simulink model "simple_walk_3d_with_feet"  (R2015a)
settings: Solver=ode23t  StartTime=0.0  StopTime=t_end  FixedStep=0.001
InitFcn:
  | colors
  | simulation_params
  | mechanical_params
StartFcn:
  | tic
StopFcn:
  | stopscript
values from neighbouring files (symbols this model uses):
  A_lpf_velocity = 1 + B1_lpf_velocity + B2_lpf_velocity    [simulation_params.m]
  ankle_stiffness = 1/2*pi    (= 1.57079632679)    [mechanical_params.m]
  B1_lpf_velocity = -2*exp(-lpf_damping*fcut_velocity*sample_time)*cos(fcut_velocity*sample_time*sqrt(1-lpf_damping^2))    [simulation_params.m]
  B2_lpf_velocity = exp(-2*lpf_damping*fcut_velocity*sample_time)    [simulation_params.m]
  b_hmotor = 0    [mechanical_params.m]
  b_leg_spring = 0.075*sqrt(k_leg_spring*0.5*.25^2)    [mechanical_params.m]
  b_rotor = 0*60/(2*pi)*9.725e-5    (= 0)    [mechanical_params.m]
  breakaway_friction = [25 25 25 25]    [mechanical_params.m]
  coulomb_friction = [20 20 20 20]    [mechanical_params.m]
  d_com = (d_hip_com_to_torso_com*m_torso)/(m_torso + num_legs*m_hshaft)    [mechanical_params.m]
  delta_phi_max = 160*pi/180    (= 2.79252680319)    [mechanical_params.m]
  delta_phi_min = 25.5*pi/180    (= 0.445058959259)    [mechanical_params.m]
  friction_linear_zone = [0.5 0.5 0.5 0.5].*pi/180    [mechanical_params.m]
  g = 9.81    [mechanical_params.m]
  HIP_MTR_MAX_TORQUE = max_current_hip*Kt_hip*N_h    (= 629.28)    [mechanical_params.m]
  initial_dx = 0    [mechanical_params.m]
  initial_hip_roll = -0.15    [mechanical_params.m]
  initial_pitch_joint_height = initial_com_height + boom_mount_to_com    [mechanical_params.m]
  initial_torso_pitch = 0*pi/180    (= 0)    [mechanical_params.m]
  initial_torso_roll = 0*pi/180    (= 0)    [mechanical_params.m]
  initial_torso_yaw = 0*pi/180    (= 0)    [mechanical_params.m]
  k_gx = m_total*g/0.005    (= 114164.30664)    [mechanical_params.m]
  k_gy = m_total*g/0.005    (= 114164.30664)    [mechanical_params.m]
  k_leg_spring = 2950    [mechanical_params.m]
  k_phi = 5000    [mechanical_params.m]
  Kb_leg = 0.121    [mechanical_params.m]
  Kt_leg = 0.121    [mechanical_params.m]
  L_leg = 0.102e-3    (= 0.000102)    [mechanical_params.m]
  l_lowerleg = 0.49    [mechanical_params.m]
  l_seg = 0.5    [mechanical_params.m]
  LEG_MTR_MAX_TORQUE = max_current_leg * Kt_leg * N    (= 1210)    [mechanical_params.m]
  lowerleg_12 = 0.40    (= 0.4)    [mechanical_params.m]
  m_fblink = 0.46    [mechanical_params.m]
  m_foot = 0.0857    [mechanical_params.m]
  m_hshaft = 18    [mechanical_params.m]
  m_lowerleg = 0.4438    [mechanical_params.m]
  m_output_gear = 1e-5    (= 1e-05)    [mechanical_params.m]
  m_rotor = 1e-5    (= 1e-05)    [mechanical_params.m]
  m_shin = 0.75    [mechanical_params.m]
  m_thigh = 0.69    [mechanical_params.m]
  m_torso = 17.5    [mechanical_params.m]
  m_total = num_legs*(m_hshaft + m_thigh + m_lowerleg + m_shin + m_fblink + 2*m_gearing) + m_torso    (= 58.18772)    [mechanical_params.m]
  m_virtual_gear = 1e-5    (= 1e-05)    [mechanical_params.m]
  max_current_leg = 200    [mechanical_params.m]
  max_voltage_leg = 50    [mechanical_params.m]
  mu_hmotor = 0.90    (= 0.9)    [mechanical_params.m]
  mu_motor = 0.85    [mechanical_params.m]
  mu_slide = 0.8    [mechanical_params.m]
  mu_stick = 0.9    [mechanical_params.m]
  N = 50    [mechanical_params.m]
  N_h = r_hip_shaft / r_hip_gearhead    (= 57)    [mechanical_params.m]
  output_sample_time = 1/30    (= 0.0333333333333)    [simulation_params.m]
  phi_max_collision = -5*pi/180    (= -0.0872664625997)    [mechanical_params.m]
  phi_roll_max = pi + 16*pi/180    (= 3.42084533391)    [mechanical_params.m]
  phi_roll_min = pi - 9*pi/180    (= 2.98451302091)    [mechanical_params.m]
  phi_shin_max = 3*pi/2 + 17.5*pi/180    (= 5.01782159948)    [mechanical_params.m]
  phi_shin_min = pi - 45*pi/180    (= 2.35619449019)    [mechanical_params.m]
  phi_thigh_max = pi + 45*pi/180    (= 3.92699081699)    [mechanical_params.m]
  phi_thigh_min = pi/2 - 17.5*pi/180    (= 1.2653637077)    [mechanical_params.m]
  r_hip_gearhead = 0.009525    [mechanical_params.m]
  r_hip_shaft = 0.542925    [mechanical_params.m]
  R_leg = 0.052    [mechanical_params.m]
  r_rotor = 0.001    [mechanical_params.m]
  r_virtual_gear = N*r_rotor    (= 0.05)    [mechanical_params.m]
  s = (clamp(f, tl, tu) - tl)/(tu - tl)    [controller.m]
  sample_time = 1/sample_freq    (= 0.001)    [simulation_params.m]
  shin_12 = 0.40    (= 0.4)    [mechanical_params.m]
  shin_initial_l = initial_l_leg_angle + acos(initial_l_leg_length)    [mechanical_params.m]
  shin_initial_r = initial_r_leg_angle + acos(initial_r_leg_length)    [mechanical_params.m]
  thigh_initial_l = initial_l_leg_angle - acos(initial_l_leg_length)    [mechanical_params.m]
  thigh_initial_r = initial_r_leg_angle - acos(initial_r_leg_length)    [mechanical_params.m]
  v_gx_max = 0.03    [mechanical_params.m]
  v_gy_max = 0.03    [mechanical_params.m]
  v_phi_max = 1/60    (= 0.0166666666667)    [mechanical_params.m]
  viscous_friction = [0.001 0.001 0.001 0.001]    [mechanical_params.m]
  vLimit = 0.01    [mechanical_params.m]
undefined symbols (not defined in the file or in its folder): fblink_color_d, floor_color_d, foot_color_d, hshaft_color_d, lowerleg_color_d, rad, sgn, shin_color_d, t_friction, thigh_color_d, torso_color_d, X, Y, Z
libraries: sm_lib x177, nesl_utility x130, simulink x57, fl_lib x16, simulink_extras x4, mblibv1 x2, commnoisgen2 x1, vrlib x1
(part 4 of 8)

== system simple_walk_3d_with_feet/Mechanical Simulation Layer/L Back Ground Contact/Ground Friction Model ==
  note: Normal Ground Stiction Model
  note: Transverse Ground Friction Model
  delta normal [m] : Inport
  vnormal [m/s] : Inport  Port=2
  x [m] : Inport  Port=3
  vx [m/s] : Inport  Port=4
  y [m] : Inport  Port=5
  vy [m/s] : Inport  Port=6
  Contact! : EnablePort  StatesWhenEnabling=reset
  Data Type Conversion : DataTypeConversion  OutDataTypeStr=double
  Friction Switch : Subsystem
  Gain3 : Gain  Gain=k_gy
  Gain4 : Gain  Gain=1/v_gy_max
  Logical Operator : Logic  Operator=NOT  AllPortsSameDT=off  OutDataTypeStr=boolean
  Mux1 : Mux  Inputs=2
  Sum1 : Sum
  Sum2 : Sum
  normal-Axis Ground Force : Fcn  Expr="- u(1)  *  (1-u(2)) * (u(2)<1)"
  t-Axis Kinetic Friction Model : Subsystem
  t-Axis Static Friction Model : Subsystem
  FxFriction [N] : Outport  OutputWhenDisabled=reset  InitialOutput=0
      settings: AttributesFormatString=initial = '%<InitialOutput>'\nwhen\ndisabled\n'%<OutputWhenDisabled>'
  FyFriction [N] : Outport  Port=2  OutputWhenDisabled=reset  InitialOutput=0
      settings: AttributesFormatString=initial = '%<InitialOutput>'\nwhen\ndisabled\n'%<OutputWhenDisabled>'
  Fn_Ground[N] : Outport  Port=3  OutputWhenDisabled=reset  InitialOutput=0
      settings: AttributesFormatString=initial = '%<InitialOutput>'\nwhen disabled = '%<OutputWhenDisabled>'
  Stiction! : Outport  Port=4  OutputWhenDisabled=reset  InitialOutput=0
      settings: AttributesFormatString=initial = '%<InitialOutput>'\nwhen\ndisabled\n'%<OutputWhenDisabled>'
  wires:
  Data Type Conversion/1 -> Stiction!/1
  vy [m/s]/1 -> t-Axis Static Friction Model/5(vel_y [m/s]), t-Axis Kinetic Friction Model/4(vel_y [m/s])
  y [m]/1 -> t-Axis Kinetic Friction Model/3(pos_y [m]), t-Axis Static Friction Model/4(pos_y [m])
  t-Axis Kinetic Friction Model/2(posFP_y [m]) -> t-Axis Static Friction Model/7(posFP_y [m])
  Sum2/1 -> FyFriction [N]/1
  t-Axis Kinetic Friction Model/5(Fy_Slide [N]) -> Sum2/2
  t-Axis Static Friction Model/1(Fy_Stick [N]) -> Sum2/1
  Gain4/1 -> Mux1/2
  Gain3/1 -> Mux1/1
  Mux1/1 -> normal-Axis Ground Force/1
  Logical Operator/1 -> t-Axis Kinetic Friction Model/Enable
  t-Axis Kinetic Friction Model/3(Stiction!) -> Friction Switch/2(Stick!)
  t-Axis Static Friction Model/3(Sliding!) -> Friction Switch/1(Slide!)
  Friction Switch/1(Stiction) -> t-Axis Static Friction Model/Enable, Logical Operator/1, Data Type Conversion/1
  Sum1/1 -> FxFriction [N]/1
  t-Axis Static Friction Model/2(Fx_Stick [N]) -> Sum1/1
  t-Axis Kinetic Friction Model/4(Fx_Slide [N]) -> Sum1/2
  t-Axis Kinetic Friction Model/1(posFP_x [m]) -> t-Axis Static Friction Model/6(posFP_x [m])
  vx [m/s]/1 -> t-Axis Static Friction Model/3(vel_x [m/s]), t-Axis Kinetic Friction Model/2(vel_x [m/s])
  x [m]/1 -> t-Axis Static Friction Model/2(pos_x [m]), t-Axis Kinetic Friction Model/1(pos_x [m])
  vnormal [m/s]/1 -> Gain4/1
  delta normal [m]/1 -> Gain3/1
  normal-Axis Ground Force/1 -> Fn_Ground[N]/1, t-Axis Kinetic Friction Model/5(F_Normal [N]), t-Axis Static Friction Model/1(F_Normal [N])

== system simple_walk_3d_with_feet/Mechanical Simulation Layer/L Front Ground Contact/Ground Friction Model ==
  note: Transverse Ground Friction Model
  note: Normal Ground Stiction Model
  delta normal [m] : Inport
  vnormal [m/s] : Inport  Port=2
  x [m] : Inport  Port=3
  vx [m/s] : Inport  Port=4
  y [m] : Inport  Port=5
  vy [m/s] : Inport  Port=6
  Contact! : EnablePort  StatesWhenEnabling=reset
  Data Type Conversion : DataTypeConversion  OutDataTypeStr=double
  Friction Switch : Subsystem
  Gain3 : Gain  Gain=k_gy
  Gain4 : Gain  Gain=1/v_gy_max
  Logical Operator : Logic  Operator=NOT  AllPortsSameDT=off  OutDataTypeStr=boolean
  Mux1 : Mux  Inputs=2
  Sum1 : Sum
  Sum2 : Sum
  normal-Axis Ground Force : Fcn  Expr="- u(1)  *  (1-u(2)) * (u(2)<1)"
  t-Axis Kinetic Friction Model : Subsystem
  t-Axis Static Friction Model : Subsystem
  FxFriction [N] : Outport  OutputWhenDisabled=reset  InitialOutput=0
      settings: AttributesFormatString=initial = '%<InitialOutput>'\nwhen\ndisabled\n'%<OutputWhenDisabled>'
  FyFriction [N] : Outport  Port=2  OutputWhenDisabled=reset  InitialOutput=0
      settings: AttributesFormatString=initial = '%<InitialOutput>'\nwhen\ndisabled\n'%<OutputWhenDisabled>'
  Fn_Ground[N] : Outport  Port=3  OutputWhenDisabled=reset  InitialOutput=0
      settings: AttributesFormatString=initial = '%<InitialOutput>'\nwhen disabled = '%<OutputWhenDisabled>'
  Stiction! : Outport  Port=4  OutputWhenDisabled=reset  InitialOutput=0
      settings: AttributesFormatString=initial = '%<InitialOutput>'\nwhen\ndisabled\n'%<OutputWhenDisabled>'
  wires:
  normal-Axis Ground Force/1 -> t-Axis Static Friction Model/1(F_Normal [N]), t-Axis Kinetic Friction Model/5(F_Normal [N]), Fn_Ground[N]/1
  delta normal [m]/1 -> Gain3/1
  vnormal [m/s]/1 -> Gain4/1
  x [m]/1 -> t-Axis Kinetic Friction Model/1(pos_x [m]), t-Axis Static Friction Model/2(pos_x [m])
  vx [m/s]/1 -> t-Axis Kinetic Friction Model/2(vel_x [m/s]), t-Axis Static Friction Model/3(vel_x [m/s])
  t-Axis Kinetic Friction Model/1(posFP_x [m]) -> t-Axis Static Friction Model/6(posFP_x [m])
  t-Axis Kinetic Friction Model/4(Fx_Slide [N]) -> Sum1/2
  t-Axis Static Friction Model/2(Fx_Stick [N]) -> Sum1/1
  Sum1/1 -> FxFriction [N]/1
  Friction Switch/1(Stiction) -> Data Type Conversion/1, Logical Operator/1, t-Axis Static Friction Model/Enable
  t-Axis Static Friction Model/3(Sliding!) -> Friction Switch/1(Slide!)
  t-Axis Kinetic Friction Model/3(Stiction!) -> Friction Switch/2(Stick!)
  Logical Operator/1 -> t-Axis Kinetic Friction Model/Enable
  Mux1/1 -> normal-Axis Ground Force/1
  Gain3/1 -> Mux1/1
  Gain4/1 -> Mux1/2
  t-Axis Static Friction Model/1(Fy_Stick [N]) -> Sum2/1
  t-Axis Kinetic Friction Model/5(Fy_Slide [N]) -> Sum2/2
  Sum2/1 -> FyFriction [N]/1
  t-Axis Kinetic Friction Model/2(posFP_y [m]) -> t-Axis Static Friction Model/7(posFP_y [m])
  y [m]/1 -> t-Axis Static Friction Model/4(pos_y [m]), t-Axis Kinetic Friction Model/3(pos_y [m])
  vy [m/s]/1 -> t-Axis Kinetic Friction Model/4(vel_y [m/s]), t-Axis Static Friction Model/5(vel_y [m/s])
  Data Type Conversion/1 -> Stiction!/1

== system simple_walk_3d_with_feet/Mechanical Simulation Layer/L Hip Shaft/Frame Data ==
  Kinematic Data : ToWorkspace  VariableName=l_hip_out  SampleTime=output_sample_time
      settings: Save2DSignal=2-D array (concatenate along first dimension)
  Mux : Mux
  PS-Simulink Converter{,1..3} (4 alike) : nesl_utility/PS-Simulink Converter  PhysicalDomain=network_engine_domain  SubClassName=ps_output  LeftPortType=input  RightPortType=output  PseudoPeriodic=off  Frequencies=[]  Unit=1  AffineConversion=off
  Transform Sensor : sm_lib/Frames and Transforms/Transform Sensor  MeasurementFrame=World  SenseAngle=off  SenseAxis=off  SenseAngle1=off  SenseAngle2=off  SenseAngle3=off  SenseQ=on  SenseR=off  SenseOmegaX=off  SenseOmegaY=off  SenseOmegaZ=off  SenseOmega1=off  SenseOmega2=off  SenseOmega3=off  SenseQDot=off  SenseRDot=off  SenseAlphaX=off  SenseAlphaY=off  SenseAlphaZ=off  SenseAlpha1=off  SenseAlpha2=off  SenseAlpha3=off  SenseQDDot=off  SenseRDDot=off  SenseX=on  SenseY=on  SenseZ=on  SenseRad=off  SenseAzim=off  SenseDist=off  SenseInc=off  SenseXDot=off  SenseYDot=off  SenseZDot=off  SenseRadDot=off  SenseAzimDot=off  SenseDistDot=off  SenseIncDot=off  SenseXDDot=off  SenseYDDot=off  SenseZDDot=off  SenseRadDDot=off  SenseAzimDDot=off  SenseDistDDot=off  SenseIncDDot=off  BlockFunction=simmechanics.library.frames_transforms.transform_sensor
  World Frame : sm_lib/Frames and Transforms/World Frame  BlockFunction=simmechanics.library.frames_transforms.world_frame
  Frame : PMIOPort  Port=1  Side=Left
  wires:
  Mux/1 -> Kinematic Data/1
  PS-Simulink Converter/1 -> Mux/1
  PS-Simulink Converter1/1 -> Mux/2
  PS-Simulink Converter2/1 -> Mux/3
  PS-Simulink Converter3/1 -> Mux/4
  connections:
  PS-Simulink Converter3/LConn1 -- Transform Sensor/RConn5
  PS-Simulink Converter2/LConn1 -- Transform Sensor/RConn4
  PS-Simulink Converter1/LConn1 -- Transform Sensor/RConn3
  PS-Simulink Converter/LConn1 -- Transform Sensor/RConn2
  Transform Sensor/RConn1 -- Frame/RConn1
  Transform Sensor/LConn1 -- World Frame/RConn1

== system simple_walk_3d_with_feet/Mechanical Simulation Layer/L Leg/Angle Range Map ==
  "[-pi, pi]" : Inport
  Constant : Constant  Value=2*pi
  Sum3 : Sum  Inputs=|++
  Switch : Switch  ZeroCross=off
  "[0,2*pi]" : Outport
  wires:
  "[-pi, pi]"/1 -> Sum3/1, Switch/1, Switch/2
  Sum3/1 -> Switch/3
  Constant/1 -> Sum3/2
  Switch/1 -> "[0,2*pi]"/1

== system simple_walk_3d_with_feet/Mechanical Simulation Layer/L Leg/Angle Range Map1 ==
  "[-pi, pi]" : Inport
  Constant : Constant  Value=2*pi
  Sum3 : Sum  Inputs=|++
  Switch : Switch  ZeroCross=off
  "[0,2*pi]" : Outport
  wires:
  Switch/1 -> "[0,2*pi]"/1
  Constant/1 -> Sum3/2
  Sum3/1 -> Switch/3
  "[-pi, pi]"/1 -> Switch/2, Switch/1, Sum3/1

== system simple_walk_3d_with_feet/Mechanical Simulation Layer/L Leg/Four Bar Link ==
  CS1 to CS2 : sm_lib/Frames and Transforms/Rigid Transform  TranslationMethod=Cartesian  TranslationLengthUnit=m  TranslationStandardAxis=+Z  TranslationStandardOffset=0  TranslationCartesianOffset=[0 -l_seg 0]  TranslationROffset=0  TranslationROffsetUnits=m  TranslationZOffset=0  TranslationZOffsetUnits=m  TranslationThetaOffset=0  TranslationThetaOffsetUnits=deg  RotationMethod=None  RotationAngleUnits=deg  RotationStandardAxis=+Z  RotationAngle=0  RotationArbitraryAxis=[0 0 1]  FollAlignAxisA=+X  BaseAlignAxisA=+Y  FollAlignAxisB=+Y  BaseAlignAxisB=+Z  RotationMatrix=[1 0 0; 0 1 0; 0 0 1]  BlockFunction=simmechanics.library.frames_transforms.rigid_transform
  Frame Data : Subsystem
  Solid : sm_lib/Body Elements/Solid  InertiaType=Custom  Mass=m_fblink  MassUnits=kg  CenterOfMass=com_fblink  CenterOfMassUnits=m  MomentsOfInertia=i_fblink_moments  MomentsOfInertiaUnits=kg*m^2  ProductsOfInertia=i_fblink_products  ProductsOfInertiaUnits=kg*m^2  DensityBased=on  Density=1000  DensityUnits=kg/(m^3)  GraphicType=FromGeometry  MarkerShape=Sphere  MarkerSize=10  MarkerSizeUnits=m  GraphicVisPropType=AdvancedVisualProperties  GraphicDiffuseColor=fblink_color_d  GraphicSpecularColor=[1 1 1 1]  GraphicAmbientColor=[fblink_color_d/2 1]  GraphicEmissiveColor=[0 0 0 1]  GraphicShininess=128  GraphicOpacity=1.0  GeometryShape=FromFile  RectangleSize=[1 1]  RectangleSizeUnits=m  BrickDimensions=[0.1 l_seg 0.1]  BrickDimensionUnits=m  CylinderRadius=l_rad  CylinderRadiusUnits=m  CylinderLength=l_seg  CylinderLengthUnits=m  SphereRadius=1  SphereRadiusUnits=m  EllipsoidRadii=[1 1 1]  EllipsoidRadiiUnits=m  ExtrusionCrossSection=[1 1; -1 1; -1 -1; 1 -1]  ExtrusionCrossSectionUnits=m  ExtrusionLength=1  ExtrusionLengthUnits=m  PolygonNumSides=3  PolygonOuterRadius=1  PolygonOuterRadiusUnits=m  ExtGeomFileType=STL  ExtGeomFileName=four_bar_link.stl  ExtGeomFileUnits=m  RevolutionCrossSection=[1 1; 1 -1; 2 -1; 2 1]  RevolutionCrossSectionUnits=m  RevolutionExtent=Full  RevolutionAngle=180  RevolutionAngleUnits=deg  BlockFunction=simmechanics.library.body_elements.solid
  CS1 : PMIOPort  Port=1  Side=Left
  CS2 : PMIOPort  Port=2  Side=Right
  connections:
  CS2/RConn1 -- CS1 to CS2/RConn1
  Solid/RConn1 -- CS1/RConn1 -- Frame Data/LConn1 -- CS1 to CS2/LConn1

== system simple_walk_3d_with_feet/Mechanical Simulation Layer/L Leg/Lower Leg ==
  CS1 to CS2 : sm_lib/Frames and Transforms/Rigid Transform  TranslationMethod=Cartesian  TranslationLengthUnit=m  TranslationStandardAxis=+Z  TranslationStandardOffset=0  TranslationCartesianOffset=[0 -lowerleg_12 0]  TranslationROffset=0  TranslationROffsetUnits=m  TranslationZOffset=0  TranslationZOffsetUnits=m  TranslationThetaOffset=0  TranslationThetaOffsetUnits=deg  RotationMethod=None  RotationAngleUnits=deg  RotationStandardAxis=+Z  RotationAngle=45  RotationArbitraryAxis=[0 0 1]  FollAlignAxisA=+X  BaseAlignAxisA=+Y  FollAlignAxisB=+Y  BaseAlignAxisB=+Z  RotationMatrix=[1 0 0; 0 1 0; 0 0 1]  BlockFunction=simmechanics.library.frames_transforms.rigid_transform
  CS1 to CS3 : sm_lib/Frames and Transforms/Rigid Transform  TranslationMethod=Cartesian  TranslationLengthUnit=m  TranslationStandardAxis=+Z  TranslationStandardOffset=0  TranslationCartesianOffset=[0 -l_lowerleg 0]  TranslationROffset=0  TranslationROffsetUnits=m  TranslationZOffset=0  TranslationZOffsetUnits=m  TranslationThetaOffset=0  TranslationThetaOffsetUnits=deg  RotationMethod=None  RotationAngleUnits=deg  RotationStandardAxis=+Y  RotationAngle=-20  RotationArbitraryAxis=[0 0 1]  FollAlignAxisA=+X  BaseAlignAxisA=+Y  FollAlignAxisB=+Y  BaseAlignAxisB=+Z  RotationMatrix=[1 0 0; 0 1 0; 0 0 1]  BlockFunction=simmechanics.library.frames_transforms.rigid_transform
  Frame Data : Subsystem
  Solid : sm_lib/Body Elements/Solid  InertiaType=Custom  Mass=m_lowerleg  MassUnits=kg  CenterOfMass=com_lowerleg  CenterOfMassUnits=m  MomentsOfInertia=i_lowerleg_moments  MomentsOfInertiaUnits=kg*m^2  ProductsOfInertia=i_lowerleg_products  ProductsOfInertiaUnits=kg*m^2  DensityBased=on  Density=1000  DensityUnits=kg/(m^3)  GraphicType=FromGeometry  MarkerShape=Sphere  MarkerSize=10  MarkerSizeUnits=m  GraphicVisPropType=AdvancedVisualProperties  GraphicDiffuseColor=lowerleg_color_d  GraphicSpecularColor=[1 1 1 1]  GraphicAmbientColor=[lowerleg_color_d/2 1]  GraphicEmissiveColor=[0 0 0 1]  GraphicShininess=128  GraphicOpacity=1.0  GeometryShape=FromFile  RectangleSize=[1 1]  RectangleSizeUnits=m  BrickDimensions=[0.1 l_seg 0.1]  BrickDimensionUnits=m  CylinderRadius=l_rad  CylinderRadiusUnits=m  CylinderLength=l_seg  CylinderLengthUnits=m  SphereRadius=1  SphereRadiusUnits=m  EllipsoidRadii=[1 1 1]  EllipsoidRadiiUnits=m  ExtrusionCrossSection=[1 1; -1 1; -1 -1; 1 -1]  ExtrusionCrossSectionUnits=m  ExtrusionLength=1  ExtrusionLengthUnits=m  PolygonNumSides=3  PolygonOuterRadius=1  PolygonOuterRadiusUnits=m  ExtGeomFileType=STL  ExtGeomFileName=lower_leg_two_point.stl  ExtGeomFileUnits=m  RevolutionCrossSection=[1 1; 1 -1; 2 -1; 2 1]  RevolutionCrossSectionUnits=m  RevolutionExtent=Full  RevolutionAngle=180  RevolutionAngleUnits=deg  BlockFunction=simmechanics.library.body_elements.solid
  CS1 : PMIOPort  Port=1  Side=Left
  CS2 : PMIOPort  Port=2  Side=Right
  CS3 : PMIOPort  Port=3  Side=Right
  connections:
  CS3/RConn1 -- CS1 to CS3/RConn1
  Frame Data/LConn1 -- CS1 to CS3/LConn1 -- CS1 to CS2/LConn1 -- Solid/RConn1 -- CS1/RConn1
  CS2/RConn1 -- CS1 to CS2/RConn1

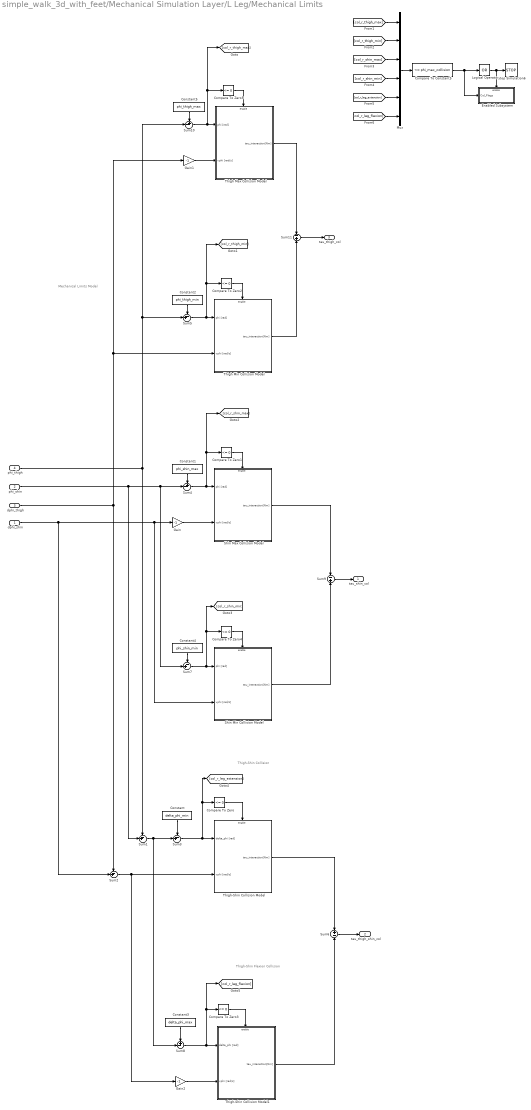
== system simple_walk_3d_with_feet/Mechanical Simulation Layer/L Leg/Mechanical Limits ==
  note: Thigh-Shin Flexion Collision
  note: Thigh-Shin Collision
  note: Mechanical Limits Model
  dphi_shin : Inport
  phi_shin : Inport  Port=2
  dphi_thigh : Inport  Port=3
  phi_thigh : Inport  Port=4
  Compare To Constant5 : simulink/Logic and Bit Operations/Compare To Constant  relop=<=  const=phi_max_collision  OutDataTypeStr=boolean  ZeroCross=off
  Compare To Zero{,1..5} (6 alike) : simulink/Logic and Bit Operations/Compare To Zero  relop=<=  OutDataTypeStr=boolean  ZeroCross=off
  Constant : Constant  Value=delta_phi_min
  Constant1 : Constant  Value=phi_shin_max
  Constant2 : Constant  Value=phi_thigh_min
  Constant3 : Constant  Value=delta_phi_max
  Constant4 : Constant  Value=phi_shin_min
  Constant5 : Constant  Value=phi_thigh_max
  Enabled Subsystem : Subsystem  TreatAsAtomicUnit=on
  Gain : Gain  Gain=-1
  Gain1 : Gain  Gain=-1
  Gain2 : Gain  Gain=-1
  Logical Operator : Logic  Operator=OR  Inputs=1  AllPortsSameDT=off  OutDataTypeStr=boolean
  Mux : Mux  Inputs=6
  Shin Max Collision Model : Subsystem
  Shin Min Collision Model : Subsystem
  Stop Simulation6 : Stop
  Sum{1..3,5,7} (5 alike) : Sum  Inputs=-+|
  Sum10 : Sum  Inputs=+-|
  Sum11 : Sum  Inputs=-|+
  Sum4 : Sum  Inputs=+-|
  Sum6 : Sum  Inputs=+|-
  Sum8 : Sum  Inputs=+-|
  Sum9 : Sum  Inputs=-|+
  Thigh Max Collision Model : Subsystem
  Thigh Min Collision Model : Subsystem
  Thigh-Shin Collision Model : Subsystem
  Thigh-Shin Collision Model1 : Subsystem
  tau_shin_col : Outport
  tau_thigh_shin_col : Outport  Port=2
  tau_thigh_col : Outport  Port=3
  wires:
  Compare To Constant5/1 -> Logical Operator/1, Enabled Subsystem/1(Col_Flags)
  Sum4/1 -> Shin Max Collision Model/1(phi [rad]), Compare To Zero1/1, [col_r_shin_max]
  Sum10/1 -> [col_r_thigh_max], Compare To Zero5/1, Thigh Max Collision Model/1(phi [rad])
  Logical Operator/1 -> Enabled Subsystem/Enable, Stop Simulation6/1
  Mux/1 -> Compare To Constant5/1
  [col_r_leg_flexion] -> Mux/6
  [col_r_leg_extension] -> Mux/5
  [col_r_shin_min] -> Mux/4
  [col_r_shin_max] -> Mux/3
  [col_r_thigh_min] -> Mux/2
  [col_r_thigh_max] -> Mux/1
  Thigh Max Collision Model/1(tau_interaction[Nm]) -> Sum11/1
  Gain1/1 -> Thigh Max Collision Model/2(vphi [rad/s])
  Thigh Min Collision Model/1(tau_interaction[Nm]) -> Sum11/2
  Sum11/1 -> tau_thigh_col/1
  Compare To Zero5/1 -> Thigh Max Collision Model/Enable
  Constant5/1 -> Sum10/1
  Sum6/1 -> tau_thigh_shin_col/1
  Shin Min Collision Model/1(tau_interaction[Nm]) -> Sum9/2
  Shin Max Collision Model/1(tau_interaction[Nm]) -> Sum9/1
  Sum9/1 -> tau_shin_col/1
  dphi_shin/1 -> Shin Min Collision Model/2(vphi [rad/s]), Gain/1, Sum2/2
  Sum7/1 -> Shin Min Collision Model/1(phi [rad]), Compare To Zero4/1, [col_r_shin_min]
  Constant4/1 -> Sum7/1
  Compare To Zero4/1 -> Shin Min Collision Model/Enable
  Gain2/1 -> Thigh-Shin Collision Model1/2(vphi [rad/s])
  Thigh-Shin Collision Model1/1(tau_interaction[Nm]) -> Sum6/2
  Thigh-Shin Collision Model/1(tau_interaction[Nm]) -> Sum6/1
  Sum8/1 -> Thigh-Shin Collision Model1/1(delta_phi [rad]), Compare To Zero3/1, [col_r_leg_flexion]
  Constant3/1 -> Sum8/1
  Compare To Zero3/1 -> Thigh-Shin Collision Model1/Enable
  Compare To Zero2/1 -> Thigh Min Collision Model/Enable
  Gain/1 -> Shin Max Collision Model/2(vphi [rad/s])
  Sum5/1 -> Thigh Min Collision Model/1(phi [rad]), Compare To Zero2/1, [col_r_thigh_min]
  Constant2/1 -> Sum5/1
  dphi_thigh/1 -> Sum2/1, Gain1/1, Thigh Min Collision Model/2(vphi [rad/s])
  phi_thigh/1 -> Sum1/1, Sum5/2, Sum10/2
  Constant1/1 -> Sum4/1
  Compare To Zero1/1 -> Shin Max Collision Model/Enable
  Sum3/1 -> Thigh-Shin Collision Model/1(delta_phi [rad]), Compare To Zero/1, [col_r_leg_extension]
  Constant/1 -> Sum3/1
  Sum2/1 -> Thigh-Shin Collision Model/2(vphi [rad/s]), Gain2/1
  phi_shin/1 -> Sum4/2, Sum7/2, Sum1/2
  Sum1/1 -> Sum3/2, Sum8/2
  Compare To Zero/1 -> Thigh-Shin Collision Model/Enable

== system simple_walk_3d_with_feet/Mechanical Simulation Layer/L Leg/Shin ==
  CS1 to CS2 : sm_lib/Frames and Transforms/Rigid Transform  TranslationMethod=Cartesian  TranslationLengthUnit=m  TranslationStandardAxis=+Z  TranslationStandardOffset=0  TranslationCartesianOffset=[0 -shin_12 0]  TranslationROffset=0  TranslationROffsetUnits=m  TranslationZOffset=0  TranslationZOffsetUnits=m  TranslationThetaOffset=0  TranslationThetaOffsetUnits=deg  RotationMethod=None  RotationAngleUnits=deg  RotationStandardAxis=+Z  RotationAngle=0  RotationArbitraryAxis=[0 0 1]  FollAlignAxisA=+X  BaseAlignAxisA=+Y  FollAlignAxisB=+Y  BaseAlignAxisB=+Z  RotationMatrix=[1 0 0; 0 1 0; 0 0 1]  BlockFunction=simmechanics.library.frames_transforms.rigid_transform
  Frame Data : Subsystem
  Solid : sm_lib/Body Elements/Solid  InertiaType=Custom  Mass=m_shin  MassUnits=kg  CenterOfMass=com_shin  CenterOfMassUnits=m  MomentsOfInertia=i_shin_moments  MomentsOfInertiaUnits=kg*m^2  ProductsOfInertia=i_shin_products  ProductsOfInertiaUnits=kg*m^2  DensityBased=on  Density=1000  DensityUnits=kg/(m^3)  GraphicType=FromGeometry  MarkerShape=Sphere  MarkerSize=10  MarkerSizeUnits=m  GraphicVisPropType=AdvancedVisualProperties  GraphicDiffuseColor=shin_color_d  GraphicSpecularColor=[1 1 1 1]  GraphicAmbientColor=[shin_color_d/2 1]  GraphicEmissiveColor=[0 0 0 1]  GraphicShininess=128  GraphicOpacity=1.0  GeometryShape=FromFile  RectangleSize=[1 1]  RectangleSizeUnits=m  BrickDimensions=[1 1 1]  BrickDimensionUnits=m  CylinderRadius=l_rad  CylinderRadiusUnits=m  CylinderLength=l_seg  CylinderLengthUnits=m  SphereRadius=1  SphereRadiusUnits=m  EllipsoidRadii=[1 1 1]  EllipsoidRadiiUnits=m  ExtrusionCrossSection=[1 1; -1 1; -1 -1; 1 -1]  ExtrusionCrossSectionUnits=m  ExtrusionLength=1  ExtrusionLengthUnits=m  PolygonNumSides=3  PolygonOuterRadius=1  PolygonOuterRadiusUnits=m  ExtGeomFileType=STL  ExtGeomFileName=shin.stl  ExtGeomFileUnits=m  RevolutionCrossSection=[1 1; 1 -1; 2 -1; 2 1]  RevolutionCrossSectionUnits=m  RevolutionExtent=Full  RevolutionAngle=180  RevolutionAngleUnits=deg  BlockFunction=simmechanics.library.body_elements.solid
  CS1 : PMIOPort  Port=1  Side=Left
  CS2 : PMIOPort  Port=2  Side=Right
  connections:
  CS1 to CS2/LConn1 -- CS1/RConn1 -- Frame Data/LConn1 -- Solid/RConn1
  CS2/RConn1 -- CS1 to CS2/RConn1

== system simple_walk_3d_with_feet/Mechanical Simulation Layer/L Leg/Shin SEA ==
  note: Shin SEA Mechanics
  Shin Gear Torque [Nm] : Inport
  Shin Joint [rad rad/s] : Inport  Port=2
  Demux : Demux  Outputs=2
  Gain : Gain  Gain=k_leg_spring
  Gain1 : Gain  Gain=b_leg_spring
  Initial Gear Angle : Constant  Value=shin_initial_l
  Inverse Gear Ratio2 : Gain  Gain=1/N
  Inverse Gear Ratio3 : Gain  Gain=Kt_leg
  Inverse Gear Ratio4 : Gain  Gain=1/Kt_leg
  Motor Efficiency : Gain  Gain=mu_motor
  Motor Controller : Subsystem  Commented=on
  Motor Electromagnetism : Subsystem  Commented=on
  Rotor Damping : Gain  Gain=b_rotor
  Rotor and Gearing : Subsystem
  Sum : Sum  Inputs=++|
  Sum2 : Sum  Inputs=+|-
  Sum3 : Sum  Inputs=|+-
  Sum4 : Sum  Inputs=+|-
  Sum5 : Sum  Inputs=|++
  Torque Limiter (outside) 2 : Saturate  UpperLimit=LEG_MTR_MAX_TORQUE  LowerLimit=-LEG_MTR_MAX_TORQUE  ZeroCross=off
      settings: AttributesFormatString=Hi: %<UpperLimit>\nLo: %<LowerLimit>
  Rotor Joint Conn : PMIOPort  Port=1  Side=Left
  Shin Joint Torque [Nm] : Outport
  Shin Gear [rad] : Outport  Port=2
  wires:
  Sum2/1 -> Gain/1
  Sum5/1 -> Rotor and Gearing/2(Spring Torque [Nm]), Shin Joint Torque [Nm]/1
  Sum3/1 -> Motor Efficiency/1
  Rotor Damping/1 -> Sum3/2
  Gain/1 -> Sum5/1  "tau_load"
  Gain1/1 -> Sum5/2
  Sum4/1 -> Gain1/1
  Shin Joint [rad rad/s]/1 -> Demux/1
  Demux/1 -> Sum2/2
  Demux/2 -> Sum4/2
  Inverse Gear Ratio3/1 -> Sum3/1
  Initial Gear Angle/1 -> Sum/1
  Sum/1 -> Shin Gear [rad]/1, Sum2/1
  Rotor and Gearing/1(Gearhead Position [rad]) -> Sum/2
  Rotor and Gearing/2(Gearhead Velocity [rad/s]) -> Sum4/1
  Motor Efficiency/1 -> Rotor and Gearing/1(Rotor Torque [Nm])
  Inverse Gear Ratio4/1 -> Inverse Gear Ratio3/1
  Motor Controller/1(Voltage [V]) -> Motor Electromagnetism/1(Voltage [V])
  Motor Electromagnetism/1(Current [A]) -> Motor Controller/2(Measured Current [A])
  Shin Gear Torque [Nm]/1 -> Torque Limiter (outside) 2/1
  Inverse Gear Ratio2/1 -> Inverse Gear Ratio4/1
  Rotor and Gearing/3(Rotor Velocity [rad/s]) -> Rotor Damping/1
  Torque Limiter (outside) 2/1 -> Inverse Gear Ratio2/1
  connections:
  Rotor and Gearing/LConn1 -- Rotor Joint Conn/RConn1

== system simple_walk_3d_with_feet/Mechanical Simulation Layer/L Leg/Thigh ==
  CS1 to CS2 : sm_lib/Frames and Transforms/Rigid Transform  TranslationMethod=Cartesian  TranslationLengthUnit=m  TranslationStandardAxis=+Z  TranslationStandardOffset=0  TranslationCartesianOffset=[0 -l_seg 0]  TranslationROffset=0  TranslationROffsetUnits=m  TranslationZOffset=0  TranslationZOffsetUnits=m  TranslationThetaOffset=0  TranslationThetaOffsetUnits=deg  RotationMethod=None  RotationAngleUnits=deg  RotationStandardAxis=+Z  RotationAngle=0  RotationArbitraryAxis=[0 0 1]  FollAlignAxisA=+X  BaseAlignAxisA=+Y  FollAlignAxisB=+Y  BaseAlignAxisB=+Z  RotationMatrix=[1 0 0; 0 1 0; 0 0 1]  BlockFunction=simmechanics.library.frames_transforms.rigid_transform
  Frame Data : Subsystem
  Solid : sm_lib/Body Elements/Solid  InertiaType=Custom  Mass=m_thigh  MassUnits=kg  CenterOfMass=com_thigh  CenterOfMassUnits=m  MomentsOfInertia=i_thigh_moments  MomentsOfInertiaUnits=kg*m^2  ProductsOfInertia=i_thigh_products  ProductsOfInertiaUnits=kg*m^2  DensityBased=on  Density=1000  DensityUnits=kg/(m^3)  GraphicType=FromGeometry  MarkerShape=Sphere  MarkerSize=10  MarkerSizeUnits=m  GraphicVisPropType=AdvancedVisualProperties  GraphicDiffuseColor=thigh_color_d  GraphicSpecularColor=[1 1 1 1]  GraphicAmbientColor=[thigh_color_d/2 1.0]  GraphicEmissiveColor=[0 0 0 1]  GraphicShininess=128  GraphicOpacity=1.0  GeometryShape=FromFile  RectangleSize=[1 1]  RectangleSizeUnits=m  BrickDimensions=[1 1 1]  BrickDimensionUnits=m  CylinderRadius=l_rad  CylinderRadiusUnits=m  CylinderLength=l_seg  CylinderLengthUnits=m  SphereRadius=1  SphereRadiusUnits=m  EllipsoidRadii=[1 1 1]  EllipsoidRadiiUnits=m  ExtrusionCrossSection=[1 1; -1 1; -1 -1; 1 -1]  ExtrusionCrossSectionUnits=m  ExtrusionLength=1  ExtrusionLengthUnits=m  PolygonNumSides=3  PolygonOuterRadius=1  PolygonOuterRadiusUnits=m  ExtGeomFileType=STL  ExtGeomFileName=thigh.stl  ExtGeomFileUnits=m  RevolutionCrossSection=[1 1; 1 -1; 2 -1; 2 1]  RevolutionCrossSectionUnits=m  RevolutionExtent=Full  RevolutionAngle=180  RevolutionAngleUnits=deg  BlockFunction=simmechanics.library.body_elements.solid
  CS1 : PMIOPort  Port=1  Side=Left
  CS2 : PMIOPort  Port=2  Side=Right
  connections:
  CS2/RConn1 -- CS1 to CS2/RConn1
  CS1 to CS2/LConn1 -- Solid/RConn1 -- Frame Data/LConn1 -- CS1/RConn1

== system simple_walk_3d_with_feet/Mechanical Simulation Layer/L Leg/Thigh SEA ==
  note: Thigh SEA Mechanics
  Thigh Gear Torque [Nm] : Inport
  Thigh Joint [rad rad/s] : Inport  Port=2
  Continuous Angle : mblibv1/Utilities/Continuous Angle  rad=rad  rads=rad/s
  Demux : Demux  Outputs=2
  Gain : Gain  Gain=k_leg_spring
  Gain1 : Gain  Gain=b_leg_spring
  Initial Gear Angle : Constant  Value=thigh_initial_l
  Inverse Gear Ratio1 : Gain  Gain=1/N
  Inverse Gear Ratio2 : Gain  Gain=Kt_leg
  Inverse Gear Ratio3 : Gain  Gain=1/Kt_leg
  Motor Efficiency : Gain  Gain=mu_motor
  Motor Controller : Subsystem  Commented=on
  Motor Electromagnetism : Subsystem  Commented=on
  Rotor Damping : Gain  Gain=b_rotor
  Rotor and Gearing : Subsystem
  Sum : Sum  Inputs=++|
  Sum2 : Sum  Inputs=+|-
  Sum3 : Sum  Inputs=|+-
  Sum4 : Sum  Inputs=+|-
  Sum5 : Sum  Inputs=|++
  Torque Limiter (outside) 2 : Saturate  UpperLimit=LEG_MTR_MAX_TORQUE  LowerLimit=-LEG_MTR_MAX_TORQUE  ZeroCross=off
      settings: AttributesFormatString=Hi: %<UpperLimit>\nLo: %<LowerLimit>
  Rotor Joint Conn : PMIOPort  Port=1  Side=Left
  Thigh Joint Torque [Nm] : Outport
  Thigh Gear [rad] : Outport  Port=2
  wires:
  Sum2/1 -> Gain/1
  Sum3/1 -> Motor Efficiency/1
  Rotor Damping/1 -> Sum3/2
  Gain/1 -> Sum5/1  "tau_load"
  Gain1/1 -> Sum5/2
  Sum4/1 -> Gain1/1
  Thigh Joint [rad rad/s]/1 -> Demux/1
  Demux/1 -> Sum2/2
  Demux/2 -> Sum4/2
  Inverse Gear Ratio3/1 -> Inverse Gear Ratio2/1
  Inverse Gear Ratio2/1 -> Sum3/1
  Initial Gear Angle/1 -> Sum/1
  Sum/1 -> Thigh Gear [rad]/1, Sum2/1
  Continuous Angle/1 -> Sum/2
  Rotor and Gearing/2(Gearhead Velocity [rad/s]) -> Sum4/1, Continuous Angle/2
  Rotor and Gearing/1(Gearhead Position [rad]) -> Continuous Angle/1
  Motor Controller/1(Voltage [V]) -> Motor Electromagnetism/1(Voltage [V])
  Motor Electromagnetism/1(Current [A]) -> Motor Controller/2(Measured Current [A])
  Thigh Gear Torque [Nm]/1 -> Torque Limiter (outside) 2/1
  Inverse Gear Ratio1/1 -> Inverse Gear Ratio3/1
  Sum5/1 -> Rotor and Gearing/2(Spring Torque [Nm]), Thigh Joint Torque [Nm]/1
  Motor Efficiency/1 -> Rotor and Gearing/1(Rotor Torque [Nm])
  Rotor and Gearing/3(Rotor Velocity [rad/s]) -> Rotor Damping/1
  Torque Limiter (outside) 2/1 -> Inverse Gear Ratio1/1
  connections:
  Rotor and Gearing/LConn1 -- Rotor Joint Conn/RConn1

== system simple_walk_3d_with_feet/Mechanical Simulation Layer/Left Hip Roll Joint/Mechanical Limits  ==
  vphi : Inport
  phi : Inport  Port=2
  Compare To Constant5 : simulink/Logic and Bit Operations/Compare To Constant  relop=<=  const=phi_max_collision  OutDataTypeStr=boolean  ZeroCross=off
  Compare To Zero1 : simulink/Logic and Bit Operations/Compare To Zero  relop=<=  OutDataTypeStr=boolean  ZeroCross=off
  Compare To Zero2 : simulink/Logic and Bit Operations/Compare To Zero  relop=<=  OutDataTypeStr=boolean  ZeroCross=off
  Constant1 : Constant  Value=phi_roll_min
  Constant2 : Constant  Value=phi_roll_max
  Enabled Subsystem : Subsystem  TreatAsAtomicUnit=on
  Gain2 : Gain  Gain=-1
  Logical Operator : Logic  Operator=OR  Inputs=1  AllPortsSameDT=off  OutDataTypeStr=boolean
  Mux : Mux  Inputs=2
  Roll Max Collision Model : Subsystem
  Roll Min Collision Model : Subsystem
  Stop Simulation6 : Stop
  Sum1 : Sum  Inputs=-+|
  Sum11 : Sum  Inputs=-|+
  Sum5 : Sum  Inputs=+-|
  tau_reaction : Outport
  wires:
  Gain2/1 -> Roll Max Collision Model/2(vphi [rad/s])
  vphi/1 -> Gain2/1, Roll Min Collision Model/2(vphi [rad/s])
  Roll Max Collision Model/1(tau_interaction[Nm]) -> Sum11/1
  Compare To Zero2/1 -> Roll Max Collision Model/Enable
  Sum5/1 -> Roll Max Collision Model/1(phi [rad]), Compare To Zero2/1, [col_hip_max]
  Constant2/1 -> Sum5/1
  Compare To Constant5/1 -> Logical Operator/1, Enabled Subsystem/1(Col_Flags)
  Constant1/1 -> Sum1/1
  Sum11/1 -> tau_reaction/1
  [col_hip_min] -> Mux/2
  Mux/1 -> Compare To Constant5/1
  [col_hip_max] -> Mux/1
  Logical Operator/1 -> Stop Simulation6/1, Enabled Subsystem/Enable
  phi/1 -> Sum5/2, Sum1/2
  Compare To Zero1/1 -> Roll Min Collision Model/Enable
  Roll Min Collision Model/1(tau_interaction[Nm]) -> Sum11/2
  Sum1/1 -> Roll Min Collision Model/1(phi [rad]), Compare To Zero1/1, [col_hip_min]

== system simple_walk_3d_with_feet/Mechanical Simulation Layer/R Back Ground Contact/Ground Friction Model ==
  note: Transverse Ground Friction Model
  note: Normal Ground Stiction Model
  delta normal [m] : Inport
  vnormal [m/s] : Inport  Port=2
  x [m] : Inport  Port=3
  vx [m/s] : Inport  Port=4
  y [m] : Inport  Port=5
  vy [m/s] : Inport  Port=6
  Contact! : EnablePort  StatesWhenEnabling=reset
  Data Type Conversion : DataTypeConversion  OutDataTypeStr=double
  Friction Switch : Subsystem
  Gain3 : Gain  Gain=k_gy
  Gain4 : Gain  Gain=1/v_gy_max
  Logical Operator : Logic  Operator=NOT  AllPortsSameDT=off  OutDataTypeStr=boolean
  Mux1 : Mux  Inputs=2
  Sum1 : Sum
  Sum2 : Sum
  normal-Axis Ground Force : Fcn  Expr="- u(1)  *  (1-u(2)) * (u(2)<1)"
  t-Axis Kinetic Friction Model : Subsystem
  t-Axis Static Friction Model : Subsystem
  FxFriction [N] : Outport  OutputWhenDisabled=reset  InitialOutput=0
      settings: AttributesFormatString=initial = '%<InitialOutput>'\nwhen\ndisabled\n'%<OutputWhenDisabled>'
  FyFriction [N] : Outport  Port=2  OutputWhenDisabled=reset  InitialOutput=0
      settings: AttributesFormatString=initial = '%<InitialOutput>'\nwhen\ndisabled\n'%<OutputWhenDisabled>'
  Fn_Ground[N] : Outport  Port=3  OutputWhenDisabled=reset  InitialOutput=0
      settings: AttributesFormatString=initial = '%<InitialOutput>'\nwhen disabled = '%<OutputWhenDisabled>'
  Stiction! : Outport  Port=4  OutputWhenDisabled=reset  InitialOutput=0
      settings: AttributesFormatString=initial = '%<InitialOutput>'\nwhen\ndisabled\n'%<OutputWhenDisabled>'
  wires:
  normal-Axis Ground Force/1 -> t-Axis Static Friction Model/1(F_Normal [N]), t-Axis Kinetic Friction Model/5(F_Normal [N]), Fn_Ground[N]/1
  delta normal [m]/1 -> Gain3/1
  vnormal [m/s]/1 -> Gain4/1
  x [m]/1 -> t-Axis Kinetic Friction Model/1(pos_x [m]), t-Axis Static Friction Model/2(pos_x [m])
  vx [m/s]/1 -> t-Axis Kinetic Friction Model/2(vel_x [m/s]), t-Axis Static Friction Model/3(vel_x [m/s])
  t-Axis Kinetic Friction Model/1(posFP_x [m]) -> t-Axis Static Friction Model/6(posFP_x [m])
  t-Axis Kinetic Friction Model/4(Fx_Slide [N]) -> Sum1/2
  t-Axis Static Friction Model/2(Fx_Stick [N]) -> Sum1/1
  Sum1/1 -> FxFriction [N]/1
  Friction Switch/1(Stiction) -> Data Type Conversion/1, Logical Operator/1, t-Axis Static Friction Model/Enable
  t-Axis Static Friction Model/3(Sliding!) -> Friction Switch/1(Slide!)
  t-Axis Kinetic Friction Model/3(Stiction!) -> Friction Switch/2(Stick!)
  Logical Operator/1 -> t-Axis Kinetic Friction Model/Enable
  Mux1/1 -> normal-Axis Ground Force/1
  Gain3/1 -> Mux1/1
  Gain4/1 -> Mux1/2
  t-Axis Static Friction Model/1(Fy_Stick [N]) -> Sum2/1
  t-Axis Kinetic Friction Model/5(Fy_Slide [N]) -> Sum2/2
  Sum2/1 -> FyFriction [N]/1
  t-Axis Kinetic Friction Model/2(posFP_y [m]) -> t-Axis Static Friction Model/7(posFP_y [m])
  y [m]/1 -> t-Axis Static Friction Model/4(pos_y [m]), t-Axis Kinetic Friction Model/3(pos_y [m])
  vy [m/s]/1 -> t-Axis Kinetic Friction Model/4(vel_y [m/s]), t-Axis Static Friction Model/5(vel_y [m/s])
  Data Type Conversion/1 -> Stiction!/1

== system simple_walk_3d_with_feet/Mechanical Simulation Layer/R Front Ground Contact/Ground Friction Model ==
  note: Normal Ground Stiction Model
  note: Transverse Ground Friction Model
  delta normal [m] : Inport
  vnormal [m/s] : Inport  Port=2
  x [m] : Inport  Port=3
  vx [m/s] : Inport  Port=4
  y [m] : Inport  Port=5
  vy [m/s] : Inport  Port=6
  Contact! : EnablePort  StatesWhenEnabling=reset
  Data Type Conversion : DataTypeConversion  OutDataTypeStr=double
  Friction Switch : Subsystem
  Gain3 : Gain  Gain=k_gy
  Gain4 : Gain  Gain=1/v_gy_max
  Logical Operator : Logic  Operator=NOT  AllPortsSameDT=off  OutDataTypeStr=boolean
  Mux1 : Mux  Inputs=2
  Sum1 : Sum
  Sum2 : Sum
  normal-Axis Ground Force : Fcn  Expr="- u(1)  *  (1-u(2)) * (u(2)<1)"
  t-Axis Kinetic Friction Model : Subsystem
  t-Axis Static Friction Model : Subsystem
  FxFriction [N] : Outport  OutputWhenDisabled=reset  InitialOutput=0
      settings: AttributesFormatString=initial = '%<InitialOutput>'\nwhen\ndisabled\n'%<OutputWhenDisabled>'
  FyFriction [N] : Outport  Port=2  OutputWhenDisabled=reset  InitialOutput=0
      settings: AttributesFormatString=initial = '%<InitialOutput>'\nwhen\ndisabled\n'%<OutputWhenDisabled>'
  Fn_Ground[N] : Outport  Port=3  OutputWhenDisabled=reset  InitialOutput=0
      settings: AttributesFormatString=initial = '%<InitialOutput>'\nwhen disabled = '%<OutputWhenDisabled>'
  Stiction! : Outport  Port=4  OutputWhenDisabled=reset  InitialOutput=0
      settings: AttributesFormatString=initial = '%<InitialOutput>'\nwhen\ndisabled\n'%<OutputWhenDisabled>'
  wires:
  Data Type Conversion/1 -> Stiction!/1
  vy [m/s]/1 -> t-Axis Static Friction Model/5(vel_y [m/s]), t-Axis Kinetic Friction Model/4(vel_y [m/s])
  y [m]/1 -> t-Axis Kinetic Friction Model/3(pos_y [m]), t-Axis Static Friction Model/4(pos_y [m])
  t-Axis Kinetic Friction Model/2(posFP_y [m]) -> t-Axis Static Friction Model/7(posFP_y [m])
  Sum2/1 -> FyFriction [N]/1
  t-Axis Kinetic Friction Model/5(Fy_Slide [N]) -> Sum2/2
  t-Axis Static Friction Model/1(Fy_Stick [N]) -> Sum2/1
  Gain4/1 -> Mux1/2
  Gain3/1 -> Mux1/1
  Mux1/1 -> normal-Axis Ground Force/1
  Logical Operator/1 -> t-Axis Kinetic Friction Model/Enable
  t-Axis Kinetic Friction Model/3(Stiction!) -> Friction Switch/2(Stick!)
  t-Axis Static Friction Model/3(Sliding!) -> Friction Switch/1(Slide!)
  Friction Switch/1(Stiction) -> t-Axis Static Friction Model/Enable, Logical Operator/1, Data Type Conversion/1
  Sum1/1 -> FxFriction [N]/1
  t-Axis Static Friction Model/2(Fx_Stick [N]) -> Sum1/1
  t-Axis Kinetic Friction Model/4(Fx_Slide [N]) -> Sum1/2
  t-Axis Kinetic Friction Model/1(posFP_x [m]) -> t-Axis Static Friction Model/6(posFP_x [m])
  vx [m/s]/1 -> t-Axis Static Friction Model/3(vel_x [m/s]), t-Axis Kinetic Friction Model/2(vel_x [m/s])
  x [m]/1 -> t-Axis Static Friction Model/2(pos_x [m]), t-Axis Kinetic Friction Model/1(pos_x [m])
  vnormal [m/s]/1 -> Gain4/1
  delta normal [m]/1 -> Gain3/1
  normal-Axis Ground Force/1 -> Fn_Ground[N]/1, t-Axis Kinetic Friction Model/5(F_Normal [N]), t-Axis Static Friction Model/1(F_Normal [N])

== system simple_walk_3d_with_feet/Mechanical Simulation Layer/R Hip Shaft/Frame Data ==
  Kinematic Data : ToWorkspace  VariableName=r_hip_out  SampleTime=output_sample_time
      settings: Save2DSignal=2-D array (concatenate along first dimension)
  Mux : Mux
  PS-Simulink Converter{,1..3} (4 alike) : nesl_utility/PS-Simulink Converter  PhysicalDomain=network_engine_domain  SubClassName=ps_output  LeftPortType=input  RightPortType=output  PseudoPeriodic=off  Frequencies=[]  Unit=1  AffineConversion=off
  Transform Sensor : sm_lib/Frames and Transforms/Transform Sensor  MeasurementFrame=World  SenseAngle=off  SenseAxis=off  SenseAngle1=off  SenseAngle2=off  SenseAngle3=off  SenseQ=on  SenseR=off  SenseOmegaX=off  SenseOmegaY=off  SenseOmegaZ=off  SenseOmega1=off  SenseOmega2=off  SenseOmega3=off  SenseQDot=off  SenseRDot=off  SenseAlphaX=off  SenseAlphaY=off  SenseAlphaZ=off  SenseAlpha1=off  SenseAlpha2=off  SenseAlpha3=off  SenseQDDot=off  SenseRDDot=off  SenseX=on  SenseY=on  SenseZ=on  SenseRad=off  SenseAzim=off  SenseDist=off  SenseInc=off  SenseXDot=off  SenseYDot=off  SenseZDot=off  SenseRadDot=off  SenseAzimDot=off  SenseDistDot=off  SenseIncDot=off  SenseXDDot=off  SenseYDDot=off  SenseZDDot=off  SenseRadDDot=off  SenseAzimDDot=off  SenseDistDDot=off  SenseIncDDot=off  BlockFunction=simmechanics.library.frames_transforms.transform_sensor
  World Frame : sm_lib/Frames and Transforms/World Frame  BlockFunction=simmechanics.library.frames_transforms.world_frame
  Frame : PMIOPort  Port=1  Side=Left
  wires:
  Mux/1 -> Kinematic Data/1
  PS-Simulink Converter/1 -> Mux/1
  PS-Simulink Converter1/1 -> Mux/2
  PS-Simulink Converter2/1 -> Mux/3
  PS-Simulink Converter3/1 -> Mux/4
  connections:
  PS-Simulink Converter3/LConn1 -- Transform Sensor/RConn5
  PS-Simulink Converter2/LConn1 -- Transform Sensor/RConn4
  PS-Simulink Converter1/LConn1 -- Transform Sensor/RConn3
  PS-Simulink Converter/LConn1 -- Transform Sensor/RConn2
  Transform Sensor/RConn1 -- Frame/RConn1
  Transform Sensor/LConn1 -- World Frame/RConn1

== system simple_walk_3d_with_feet/Mechanical Simulation Layer/R Leg/Angle Range Map ==
  "[-pi, pi]" : Inport
  Constant : Constant  Value=2*pi
  Sum3 : Sum  Inputs=|++
  Switch : Switch  ZeroCross=off
  "[0,2*pi]" : Outport
  wires:
  "[-pi, pi]"/1 -> Sum3/1, Switch/1, Switch/2
  Sum3/1 -> Switch/3
  Constant/1 -> Sum3/2
  Switch/1 -> "[0,2*pi]"/1

== system simple_walk_3d_with_feet/Mechanical Simulation Layer/R Leg/Angle Range Map1 ==
  "[-pi, pi]" : Inport
  Constant : Constant  Value=2*pi
  Sum3 : Sum  Inputs=|++
  Switch : Switch  ZeroCross=off
  "[0,2*pi]" : Outport
  wires:
  Switch/1 -> "[0,2*pi]"/1
  Constant/1 -> Sum3/2
  Sum3/1 -> Switch/3
  "[-pi, pi]"/1 -> Switch/2, Switch/1, Sum3/1

== system simple_walk_3d_with_feet/Mechanical Simulation Layer/R Leg/Four Bar Link ==
  CS1 to CS2 : sm_lib/Frames and Transforms/Rigid Transform  TranslationMethod=Cartesian  TranslationLengthUnit=m  TranslationStandardAxis=+Z  TranslationStandardOffset=0  TranslationCartesianOffset=[0 -l_seg 0]  TranslationROffset=0  TranslationROffsetUnits=m  TranslationZOffset=0  TranslationZOffsetUnits=m  TranslationThetaOffset=0  TranslationThetaOffsetUnits=deg  RotationMethod=None  RotationAngleUnits=deg  RotationStandardAxis=+Z  RotationAngle=0  RotationArbitraryAxis=[0 0 1]  FollAlignAxisA=+X  BaseAlignAxisA=+Y  FollAlignAxisB=+Y  BaseAlignAxisB=+Z  RotationMatrix=[1 0 0; 0 1 0; 0 0 1]  BlockFunction=simmechanics.library.frames_transforms.rigid_transform
  Frame Data : Subsystem
  Solid : sm_lib/Body Elements/Solid  InertiaType=Custom  Mass=m_fblink  MassUnits=kg  CenterOfMass=com_fblink  CenterOfMassUnits=m  MomentsOfInertia=i_fblink_moments  MomentsOfInertiaUnits=kg*m^2  ProductsOfInertia=i_fblink_products  ProductsOfInertiaUnits=kg*m^2  DensityBased=on  Density=1000  DensityUnits=kg/(m^3)  GraphicType=FromGeometry  MarkerShape=Sphere  MarkerSize=10  MarkerSizeUnits=m  GraphicVisPropType=AdvancedVisualProperties  GraphicDiffuseColor=fblink_color_d  GraphicSpecularColor=[1 1 1 1]  GraphicAmbientColor=[fblink_color_d/2 1]  GraphicEmissiveColor=[0 0 0 1]  GraphicShininess=128  GraphicOpacity=1.0  GeometryShape=FromFile  RectangleSize=[1 1]  RectangleSizeUnits=m  BrickDimensions=[0.1 l_seg 0.1]  BrickDimensionUnits=m  CylinderRadius=l_rad  CylinderRadiusUnits=m  CylinderLength=l_seg  CylinderLengthUnits=m  SphereRadius=1  SphereRadiusUnits=m  EllipsoidRadii=[1 1 1]  EllipsoidRadiiUnits=m  ExtrusionCrossSection=[1 1; -1 1; -1 -1; 1 -1]  ExtrusionCrossSectionUnits=m  ExtrusionLength=1  ExtrusionLengthUnits=m  PolygonNumSides=3  PolygonOuterRadius=1  PolygonOuterRadiusUnits=m  ExtGeomFileType=STL  ExtGeomFileName=four_bar_link.stl  ExtGeomFileUnits=m  RevolutionCrossSection=[1 1; 1 -1; 2 -1; 2 1]  RevolutionCrossSectionUnits=m  RevolutionExtent=Full  RevolutionAngle=180  RevolutionAngleUnits=deg  BlockFunction=simmechanics.library.body_elements.solid
  CS1 : PMIOPort  Port=1  Side=Left
  CS2 : PMIOPort  Port=2  Side=Right
  connections:
  CS2/RConn1 -- CS1 to CS2/RConn1
  Solid/RConn1 -- CS1/RConn1 -- Frame Data/LConn1 -- CS1 to CS2/LConn1

== system simple_walk_3d_with_feet/Mechanical Simulation Layer/R Leg/Lower Leg ==
  CS1 to CS2 : sm_lib/Frames and Transforms/Rigid Transform  TranslationMethod=Cartesian  TranslationLengthUnit=m  TranslationStandardAxis=+Z  TranslationStandardOffset=0  TranslationCartesianOffset=[0 -lowerleg_12 0]  TranslationROffset=0  TranslationROffsetUnits=m  TranslationZOffset=0  TranslationZOffsetUnits=m  TranslationThetaOffset=0  TranslationThetaOffsetUnits=deg  RotationMethod=None  RotationAngleUnits=deg  RotationStandardAxis=+Z  RotationAngle=0  RotationArbitraryAxis=[0 0 1]  FollAlignAxisA=+X  BaseAlignAxisA=+Y  FollAlignAxisB=+Y  BaseAlignAxisB=+Z  RotationMatrix=[1 0 0; 0 1 0; 0 0 1]  BlockFunction=simmechanics.library.frames_transforms.rigid_transform
  CS1 to CS3 : sm_lib/Frames and Transforms/Rigid Transform  TranslationMethod=Cartesian  TranslationLengthUnit=m  TranslationStandardAxis=+Z  TranslationStandardOffset=0  TranslationCartesianOffset=[0 -l_lowerleg 0]  TranslationROffset=0  TranslationROffsetUnits=m  TranslationZOffset=0  TranslationZOffsetUnits=m  TranslationThetaOffset=0  TranslationThetaOffsetUnits=deg  RotationMethod=None  RotationAngleUnits=deg  RotationStandardAxis=+Y  RotationAngle=20  RotationArbitraryAxis=[0 0 1]  FollAlignAxisA=+X  BaseAlignAxisA=+Y  FollAlignAxisB=+Y  BaseAlignAxisB=+Z  RotationMatrix=[1 0 0; 0 1 0; 0 0 1]  BlockFunction=simmechanics.library.frames_transforms.rigid_transform
  Frame Data : Subsystem
  Solid : sm_lib/Body Elements/Solid  InertiaType=Custom  Mass=m_lowerleg  MassUnits=kg  CenterOfMass=com_lowerleg  CenterOfMassUnits=m  MomentsOfInertia=i_lowerleg_moments  MomentsOfInertiaUnits=kg*m^2  ProductsOfInertia=i_lowerleg_products  ProductsOfInertiaUnits=kg*m^2  DensityBased=on  Density=1000  DensityUnits=kg/(m^3)  GraphicType=FromGeometry  MarkerShape=Sphere  MarkerSize=10  MarkerSizeUnits=m  GraphicVisPropType=AdvancedVisualProperties  GraphicDiffuseColor=lowerleg_color_d  GraphicSpecularColor=[1 1 1 1]  GraphicAmbientColor=[lowerleg_color_d/2 1]  GraphicEmissiveColor=[0 0 0 1]  GraphicShininess=128  GraphicOpacity=1.0  GeometryShape=FromFile  RectangleSize=[1 1]  RectangleSizeUnits=m  BrickDimensions=[0.1 l_seg 0.1]  BrickDimensionUnits=m  CylinderRadius=l_rad  CylinderRadiusUnits=m  CylinderLength=l_seg  CylinderLengthUnits=m  SphereRadius=1  SphereRadiusUnits=m  EllipsoidRadii=[1 1 1]  EllipsoidRadiiUnits=m  ExtrusionCrossSection=[1 1; -1 1; -1 -1; 1 -1]  ExtrusionCrossSectionUnits=m  ExtrusionLength=1  ExtrusionLengthUnits=m  PolygonNumSides=3  PolygonOuterRadius=1  PolygonOuterRadiusUnits=m  ExtGeomFileType=STL  ExtGeomFileName=lower_leg_two_point.stl  ExtGeomFileUnits=m  RevolutionCrossSection=[1 1; 1 -1; 2 -1; 2 1]  RevolutionCrossSectionUnits=m  RevolutionExtent=Full  RevolutionAngle=180  RevolutionAngleUnits=deg  BlockFunction=simmechanics.library.body_elements.solid
  CS1 : PMIOPort  Port=1  Side=Left
  CS2 : PMIOPort  Port=2  Side=Right
  CS3 : PMIOPort  Port=3  Side=Right
  connections:
  CS3/RConn1 -- CS1 to CS3/RConn1
  CS1 to CS3/LConn1 -- CS1 to CS2/LConn1 -- Solid/RConn1 -- Frame Data/LConn1 -- CS1/RConn1
  CS2/RConn1 -- CS1 to CS2/RConn1
